simulink model "IPD"  (R2015a)
settings: Solver=ode45  StartTime=0.0  StopTime=10  RelTol=1e-3
model workspace (MAT data in the model file):
  Var = 0.0578778135048
  Ra = 0.15
  La = 0.003
  J = 10
  K_E = 8.5
  K_T = 8.5
  T_L = 2864.873
  a_1 = 1.25
  a_0 = 1
  a_2 = 0.5
  a_3 = 0.025
  b_0 = 8.5
  b_1 = 0.176470588235
  b_2 = 0.00352941176471
  s = 0.1
settings Model: Creator=ry0  LastModifiedBy=ry0

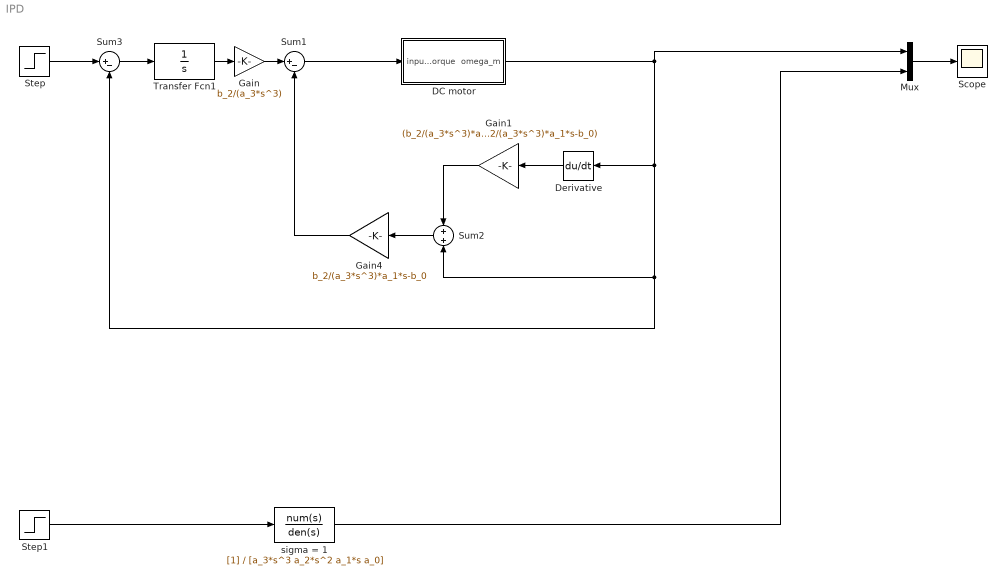
== system IPD ==
  "DC motor " : Subsystem
  Derivative : Derivative
  Gain : Gain  Gain=b_2/(a_3*s^3)
  Gain1 : Gain  Gain=(b_2/(a_3*s^3)*a_2*s^2-b_1)/(b_2/(a_3*s^3)*a_1*s-b_0)
  Gain4 : Gain  Gain=b_2/(a_3*s^3)*a_1*s-b_0
  Mux : Mux  Inputs=2
  Scope : Scope
      settings: TimeRange=12  YMin=-1250  YMax=750
  Step : Step  Time=0  After=500  SampleTime=0
  Step1 : Step  Time=0  After=500  SampleTime=0
  Sum1 : Sum  Inputs=|+-
  Sum2 : Sum
  Sum3 : Sum  Inputs=|+-
  Transfer Fcn1 : TransferFcn  Denominator=[1 0]
  sigma = 1 : TransferFcn  Denominator=[a_3*s^3 a_2*s^2 a_1*s a_0]
  wires:
  Derivative/1 -> Gain1/1
  Gain1/1 -> Sum2/1
  "DC motor "/1(omega_m) -> Mux/1, Derivative/1, Sum2/2, Sum3/2
  Sum3/1 -> Transfer Fcn1/1
  Step/1 -> Sum3/1
  Sum2/1 -> Gain4/1
  Sum1/1 -> "DC motor "/1(input torque)
  Gain4/1 -> Sum1/2
  Transfer Fcn1/1 -> Gain/1
  Gain/1 -> Sum1/1
  sigma = 1/1 -> Mux/2
  Step1/1 -> sigma = 1/1
  Mux/1 -> Scope/1

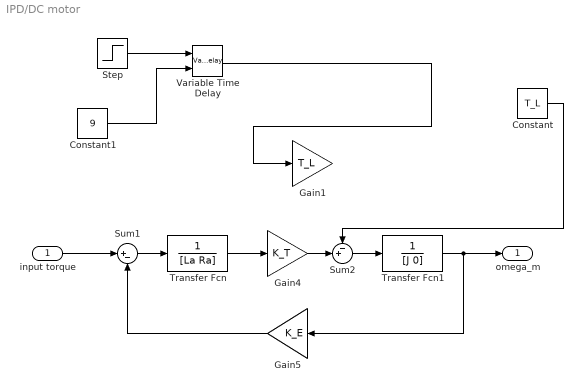
== system IPD/DC motor  ==
  input torque : Inport
  Constant : Constant  Value=T_L
  Constant1 : Constant  Value=9
  Gain1 : Gain  Gain=T_L
  Gain4 : Gain  Gain=K_T
  Gain5 : Gain  Gain=K_E
  Step : Step  SampleTime=0
  Sum1 : Sum  Inputs=|+-
  Sum2 : Sum  Inputs=-+|
  Transfer Fcn : TransferFcn  Denominator=[La Ra]
  Transfer Fcn1 : TransferFcn  Denominator=[J 0]
  Variable Time Delay : VariableTransportDelay  MaximumDelay=10
  omega_m : Outport
  wires:
  Sum1/1 -> Transfer Fcn/1
  Transfer Fcn/1 -> Gain4/1
  Gain4/1 -> Sum2/2
  Transfer Fcn1/1 -> Gain5/1, omega_m/1
  Gain5/1 -> Sum1/2
  Sum2/1 -> Transfer Fcn1/1
  input torque/1 -> Sum1/1
  Step/1 -> Variable Time Delay/1
  Constant1/1 -> Variable Time Delay/2
  Variable Time Delay/1 -> Gain1/1
  Constant/1 -> Sum2/1
